simulink model "EV_thermal_charger_2015a_jmaab_Can02"  (R2015a)
settings: Solver=ode3  StartTime=0.0  StopTime=1800  FixedStep=sampling_time  RelTol=1e-3
PreLoadFcn:
  | %run('init_setting.m')
PostLoadFcn:
  | %set_param(gcs, 'SimulationCommand', 'update');
  | %load('save_param/save_P_Charger', 'P_Charger');
  | %load('save_param/save_T_User_set_temp_degC','T_User_set_temp_degC');
  | %load('save_param/save_ENV_PNT_PTTH_Temp_add_degC','ENV_PNT_PTTH_Temp_add_degC');
  | %load('save_param/save_ENV_PNT_CABIN_Temp_add_degC','ENV_PNT_CABIN_Temp_add_degC');
  | %load('save_param/save_ENV_PNT_PHI_Sunlight_W','ENV_PNT_PHI_Sunlight_W');
  | %load('save_param/save_ENV_PNT_Outside_Temp_ini_degC','ENV_PNT_Outside_Temp_ini_degC');
StartFcn:
  | tic
StopFcn:
  | toc
  | disp(['実時間の' num2str(toc/max(tout)) '倍'])
undefined symbols (not defined in the file or in its folder): BK_PNT_Pow_UL, BK_PNT_ReGene_vel_limit_DN_kmph, BK_PNT_ReGene_vel_limit_UP_kmph, BK_PNT_Tau_brake, Brk_LL, Brk_PGain, Brk_UL, BT_PNT_Hi_C_pol_hi_batt, BT_PNT_Hi_Capa_hi_batt_F, BT_PNT_Hi_ocv_SOC_hi_batt_OCV_V_table, BT_PNT_Hi_ocv_SOC_hi_batt_OCV_V_table_x_SOC, BT_PNT_Hi_R_hi_batt_cell, BT_PNT_Hi_R_pol_hi_batt, BT_PNT_Hi_SOC_MAX_hi_batt, BT_PNT_Hi_SOC_MIN_hi_batt, BT_PNT_Hi_SOC_START_hi_batt, BT_PNT_Lo_Capa_lo_batt_F, BT_PNT_Lo_ocv_SOC_lo_batt_OCV_V_table, BT_PNT_Lo_ocv_SOC_lo_batt_OCV_V_table_x_SOC, BT_PNT_Lo_R_lo_batt_ohm, BT_PNT_Lo_SOC_MAX_lo_batt, BT_PNT_Lo_SOC_MIN_lo_batt, BT_PNT_Lo_SOC_START_lo_batt, BTTH_CNT_P_BT_Heater_W, BTTH_CNT_P_BT_Heater_W_x_BTCells_degC, BTTH_CNT_Voltage_BTFan_V, BTTH_CNT_Voltage_BTFan_V_x_BTCells_degC, BTTH_PNT_BT_Heat_Resi_KpW, BTTH_PNT_BT_Heat_Resi_KpW_x_Wind_m3ps, BTTH_PNT_BT_Heater2BTCells_Heat_Resi_KpW, BTTH_PNT_BT_Heater_Heat_Capa_JpK, BTTH_PNT_BTBlock2BTAir_Heat_Resi_KpW, BTTH_PNT_BTBlock_Heat_Capa_JpK, BTTH_PNT_BTCells2BTBlock_Heat_Resi_KpW, BTTH_PNT_BTCells_Heat_Capa_JpK, BTTH_PNT_v_BTFan_Wind_vel_mps, BTTH_PNT_v_BTFan_Wind_vel_mps_x_V_BTFan, CATH_CNT_P_Aircon_W_LL, CATH_CNT_P_Aircon_W_UL, CATH_CNT_P_Gain_Aircon, CATH_CNT_P_Gain_PTC_Heater, CATH_CNT_P_Gain_SeatHT, CATH_CNT_P_PTC_Heater, CATH_CNT_P_PTC_Heater_W_LL, CATH_CNT_P_PTC_Heater_W_UL, CATH_CNT_P_PTC_Heater_x_T_Outside_temp_degC, CATH_CNT_P_SeatHT_W_LL, CATH_CNT_P_SeatHT_W_UL, CATH_CNT_PGain_Temp_blowout, CATH_CNT_T_Aircon_Indoor_degC, CATH_CNT_T_Aircon_Indoor_degC_x_T_blowout_degC, CATH_CNT_T_PTC_Heater_degC_UL, CATH_CNT_T_SeatHT_Temp_degC, CATH_CNT_T_SeatHT_Temp_degC_x_T_blowout_degC, CATH_CNT_V_HVAC_Fan, CATH_CNT_V_HVAC_Fan_x_T_blowout_degC, CATH_CNT_V_RDFan_V, CATH_CNT_V_RDFan_x_P_Aircon_W, CATH_PNT_Air_Convection_Heat_Resi_KpW, CATH_PNT_Air_Convection_Heat_Resi_x_mps ... (+141)
undefined symbols (not defined in the file): ACC_D_Gain, ACC_I_Gain, ACC_P_Gain
libraries: METI_Lib_vehicle_model x52, simulink x35
(part 4 of 6)

== system EV_thermal_charger_2015a_jmaab_Can02/Vehicle/ELTH/ELTH_PNT/INVTH_PNT ==
  note: モーターハウジングへの熱量
  note: ヒートシンクの
      | 熱容量
  note: インバータ筐体の
      | 熱容量
  note: 冷却水からの熱量
  Temp_ini : Inport
  PHI_INV_PNT_W : Inport  Port=2
  T_ATM_PNT_INV_K : Inport  Port=3
  T_MGTH_PNT_INVTH_K : Inport  Port=4
  PHI_RD_PNT_INVTH_W : Inport  Port=5
  INVBlock2Air_Heat_Resistance : Subsystem
  INVBlock_Heat_Capacity : Subsystem
  INVHeatsink2INVBlock_Heat_Resistance : Subsystem
  INVTH_Heatsink_Heat_Capacity : Subsystem
  K->degC1 : Subsystem
  K->degC2 : Subsystem
  MG2INVBlock_Heat_Resistance : Subsystem
  T_INVHeatsink_K : Outport
  T_INVTH_PNT_K : Outport  Port=2
  PHI_INVTH_PNT_ATM_W : Outport  Port=3
  T_INVTH_PNT_RD_K : Outport  Port=4
  PHI_INVTH_PNT_MGTH_W : Outport  Port=5
  tag scope: tScope_T_INVBlock_degC=global, tScope_T_INVHeatsink_degC=global
  wires:
  INVBlock_Heat_Capacity/3(T_INVBlock1_K) -> INVHeatsink2INVBlock_Heat_Resistance/2(T_INVBlock_Resi1_K)
  INVHeatsink2INVBlock_Heat_Resistance/1(PHI_INVBlock_Resi1_W) -> INVBlock_Heat_Capacity/3(PHI_INVBlock1_W)
  INVBlock2Air_Heat_Resistance/2(PHI_INVBlock_Resi3_W) -> INVBlock_Heat_Capacity/4(PHI_INVBlock3_W)
  INVBlock_Heat_Capacity/2(T_INVBlock3_K) -> INVBlock2Air_Heat_Resistance/2(T_INVBlock_Resi3_K), K->degC1/1(K)
  INVBlock2Air_Heat_Resistance/1(PHI_INV2Air_Resi1_W) -> PHI_INVTH_PNT_ATM_W/1  "PHI_INVTH_PNT_ATM_W"
  MG2INVBlock_Heat_Resistance/1(PHI_INVBlock_Resi2_W) -> INVBlock_Heat_Capacity/1(PHI_INVBlock2_W)
  INVBlock_Heat_Capacity/1(T_INVBlock2_K) -> MG2INVBlock_Heat_Resistance/1(T_INVBlock_Resi2_K)
  T_MGTH_PNT_INVTH_K/1 -> MG2INVBlock_Heat_Resistance/2(T_MGBlock_Resi4_K)
  MG2INVBlock_Heat_Resistance/2(PHI_MGBlock_Resi4_W) -> PHI_INVTH_PNT_MGTH_W/1  "HI_INVTH_PNT_MGTH_W"
  INVTH_Heatsink_Heat_Capacity/1(T_INVTH_Heatsink1_K) -> T_INVTH_PNT_K/1  "T_INVTH_PNT_K"
  PHI_INV_PNT_W/1 -> INVTH_Heatsink_Heat_Capacity/2(PHI_INVTH_Heatsink1_W)
  T_ATM_PNT_INV_K/1 -> INVBlock2Air_Heat_Resistance/1(T_INV2Air_Resi1_K)
  INVTH_Heatsink_Heat_Capacity/3(T_INVTH_Heatsink3_K) -> T_INVTH_PNT_RD_K/1, K->degC2/1(K), T_INVHeatsink_K/1  "T_INVHeatsink_K"
  PHI_RD_PNT_INVTH_W/1 -> INVTH_Heatsink_Heat_Capacity/3(PHI_INVTH_Heatsink3_W)
  INVTH_Heatsink_Heat_Capacity/2(T_INVTH_Heatsink2_K) -> INVHeatsink2INVBlock_Heat_Resistance/1(T_INVHeatsink_Resi2_K)
  INVHeatsink2INVBlock_Heat_Resistance/2(PHI_INVHeatsink_Resi2_W) -> INVTH_Heatsink_Heat_Capacity/4(PHI_INVTH_Heatsink2_W)
  Temp_ini/1 -> INVTH_Heatsink_Heat_Capacity/1(Temp_ini), INVBlock_Heat_Capacity/2(Temp_ini)
  K->degC2/1(degC) -> [tScope_T_INVHeatsink_degC]
  K->degC1/1(degC) -> [tScope_T_INVBlock_degC]

== system EV_thermal_charger_2015a_jmaab_Can02/Vehicle/ELTH/ELTH_PNT/K->degC1 ==
  K : Inport
  Constant2 : Constant  Value=K2degC
  Sum : Sum  Inputs=++|
  degC : Outport
  wires:
  K/1 -> Sum/2
  Constant2/1 -> Sum/1
  Sum/1 -> degC/1

== system EV_thermal_charger_2015a_jmaab_Can02/Vehicle/ELTH/ELTH_PNT/K->degC3 ==
  K : Inport
  Constant2 : Constant  Value=K2degC
  Sum : Sum  Inputs=++|
  degC : Outport
  wires:
  K/1 -> Sum/2
  Constant2/1 -> Sum/1
  Sum/1 -> degC/1

== system EV_thermal_charger_2015a_jmaab_Can02/Vehicle/ELTH/ELTH_PNT/K->degC6 ==
  K : Inport
  Constant2 : Constant  Value=K2degC
  Sum : Sum  Inputs=++|
  degC : Outport
  wires:
  K/1 -> Sum/2
  Constant2/1 -> Sum/1
  Sum/1 -> degC/1

== system EV_thermal_charger_2015a_jmaab_Can02/Vehicle/ELTH/ELTH_PNT/MGTH_PNT ==
  note: モーターコイルの
      | 熱容量
  note: モーターハウジングの
      | 熱容量
  note: インバータ筐体からの熱量
  note: PTサーマルシステムへの熱量
  note: 冷却水から
      | モーターハウジングへの熱量
  note: モーターの損失が
      | コイルへの熱量
  note: モーターハウジングから大気へ
      | 放熱する熱量
  Temp_ini : Inport
  PHI_MG_PNT_W : Inport  Port=2
  T_TMTH_PNT_ELTH_K : Inport  Port=3
  T_ATM_PNT_MG_K : Inport  Port=4
  " PHI_RD_PNT_MGTH_W" : Inport  Port=5
  PHI_INVTH_PNT_MGTH_W : Inport  Port=6
  Coil_Heat_Capacity : Subsystem
  K->degC1 : Subsystem
  K->degC2 : Subsystem
  MGCoil2MGHousing_Heat_Resistance : Subsystem
  MGHousing2Air_Heat_Resistance : Subsystem
  MGHousing_Heat_Capacity : Subsystem
  PTTH2MGHousing_Heat_Resistance : Subsystem
  T_MGCoil_K : Outport
  T_MGTH_PNT_K : Outport  Port=2
  PHI_MGTH_PNT_PTTH_W : Outport  Port=3
  PHI_MGTH_PNT_ATM_W : Outport  Port=4
  T_MGTH_PNT_RD_K : Outport  Port=5
  T_MGTH_PNT_INVTH_K : Outport  Port=6
  tag scope: tScope_T_MGBlock_degC=global, tScope_T_MGCoil_degC=global
  wires:
  Coil_Heat_Capacity/2(T_MGCoil2_K) -> MGCoil2MGHousing_Heat_Resistance/1(T_MGCoil_Resi4_K), K->degC1/1(K)
  MGCoil2MGHousing_Heat_Resistance/2(PHI_MGCoil_Resi4_W) -> Coil_Heat_Capacity/3(PHI_MGCoil2_W)
  MGHousing_Heat_Capacity/5(T_MGHousing1_K) -> MGCoil2MGHousing_Heat_Resistance/2(T_MGHousing_Resi1_K)
  Coil_Heat_Capacity/1(T_MGCoil1_K) -> T_MGTH_PNT_K/1, T_MGCoil_K/1  "T_MGTH_PNT_K"
  PHI_MG_PNT_W/1 -> Coil_Heat_Capacity/2(PHI_MGCoil1_W)
  T_TMTH_PNT_ELTH_K/1 -> PTTH2MGHousing_Heat_Resistance/2(T_PTTH_Resi2_K)
  PTTH2MGHousing_Heat_Resistance/2(PHI_PTTH_Resi2_W) -> PHI_MGTH_PNT_PTTH_W/1  "PHI_MGTH_PNT_PTTH_W"
  PTTH2MGHousing_Heat_Resistance/1(PHI_MGHousing_Resi2_W) -> MGHousing_Heat_Capacity/1(PHI_MGHousing2_W)
  MGHousing_Heat_Capacity/1(T_MGHousing2_K) -> PTTH2MGHousing_Heat_Resistance/1(T_MGHousing_Resi2_K)
  T_ATM_PNT_MG_K/1 -> MGHousing2Air_Heat_Resistance/1(T_MG2Air_Resi1_K)
  MGHousing2Air_Heat_Resistance/1(PHI_MG2Air_Resi1_W) -> PHI_MGTH_PNT_ATM_W/1  "PHI_MGTH_PNT_ATM_W"
  MGHousing_Heat_Capacity/3(T_MGHousing4_K) -> T_MGTH_PNT_INVTH_K/1  "T_MGTH_PNT_INVTH_K"
  PHI_INVTH_PNT_MGTH_W/1 -> MGHousing_Heat_Capacity/3(PHI_MGHousing4_W)
  MGHousing_Heat_Capacity/4(T_MGHousing5_K) -> K->degC2/1(K), MGHousing2Air_Heat_Resistance/2(T_MGHousing_Resi5_K)
  MGHousing2Air_Heat_Resistance/2(PHI_MGHousing_Resi5_W) -> MGHousing_Heat_Capacity/6(PHI_MGHousing5_W)
  MGHousing_Heat_Capacity/2(T_MGHousing3_K) -> T_MGTH_PNT_RD_K/1  "T_MGTH_PNT_RD_K"
  " PHI_RD_PNT_MGTH_W"/1 -> MGHousing_Heat_Capacity/2(PHI_MGHousing3_W)
  Temp_ini/1 -> Coil_Heat_Capacity/1(Temp_ini), MGHousing_Heat_Capacity/4(Temp_ini)
  K->degC1/1(degC) -> [tScope_T_MGCoil_degC]
  K->degC2/1(degC) -> [tScope_T_MGBlock_degC]
  MGCoil2MGHousing_Heat_Resistance/1(PHI_MGHousing_Resi1_W) -> MGHousing_Heat_Capacity/5(PHI_MGHousing1_W)

== system EV_thermal_charger_2015a_jmaab_Can02/Vehicle/ELTH/ELTH_PNT/RD_PNT ==
  note: ラジエター～大気間
      | 熱抵抗
  note: 冷却水＋ラジエターコア
      | 熱容量
  Temp_ini : Inport
  v_VL_PNT_mps : Inport  Port=2
  V_ELTH_CNT_RDFan_V : Inport  Port=3
  V_ELTH_CNT_WP_V : Inport  Port=4
  T_ATM_PNT_RD_K : Inport  Port=5
  T_MGTH_PNT_RD_K : Inport  Port=6
  T_INVTH_PNT_RD_K : Inport  Port=7
  Add : Sum
  INV2Coolant_Heat_Resistance1 : Subsystem
  K->degC1 : Subsystem
  MG2Coolant_Heat_Resistance : Subsystem
  RDCoolant2Air_Heat_Resistance : Subsystem
  RDCoolant_Heat_Capacity : Subsystem
  RD_Core_Heat_Resi_Calc : Subsystem
  Water_Pump : Subsystem
  T_RDCoolant_K : Outport
  Heat_Resi_ELTH_PNT_AirconCore_KpW : Outport  Port=2
  PHI_RDTH_PNT_ATM_W : Outport  Port=3
  PHI_RD_PNT_MGTH_W : Outport  Port=4
  PHI_RD_PNT_INVTH_W : Outport  Port=5
  tag scope: tScope_T_RDCoolant_degC=global
  wires:
  RDCoolant_Heat_Capacity/2(T_RDCoolant1_K) -> INV2Coolant_Heat_Resistance1/3(T_Coolant_Resi_K)
  INV2Coolant_Heat_Resistance1/1(PHI_Coolant_Resi_W) -> RDCoolant_Heat_Capacity/2(PHI_RDCoolant1_W)
  RDCoolant2Air_Heat_Resistance/1(PHI_RD_Air_Resi1_W) -> PHI_RDTH_PNT_ATM_W/1  "PHI_RDTH_PNT_ATM_W"
  RDCoolant2Air_Heat_Resistance/2(PHI_RDCoolant_Resi2_W) -> RDCoolant_Heat_Capacity/3(PHI_RDCoolant2_W)
  V_ELTH_CNT_RDFan_V/1 -> RD_Core_Heat_Resi_Calc/1(ELTH_PNT_Voltage_RDFan_V)
  v_VL_PNT_mps/1 -> RD_Core_Heat_Resi_Calc/2(v_VL_PNT_mps)
  RD_Core_Heat_Resi_Calc/1("ELTH_PNT_RDCore_Heat_Resi_KpW ") -> RDCoolant2Air_Heat_Resistance/2("RD_PNT_RDCore_Heat_Resi_KpW ")
  T_ATM_PNT_RD_K/1 -> RDCoolant2Air_Heat_Resistance/1(T_RD_Air_Resi1_K)
  RDCoolant_Heat_Capacity/1(T_RDCoolant2_K) -> T_RDCoolant_K/1, K->degC1/1(K), RDCoolant2Air_Heat_Resistance/3(T_RDCoolant_Resi2_K)  "T_RDCoolant_K"
  Water_Pump/1(Qv_Coolant_m3ps) -> MG2Coolant_Heat_Resistance/2(Qv_Coolant_m3ps), INV2Coolant_Heat_Resistance1/1(Qv_Coolant_m3ps)
  T_MGTH_PNT_RD_K/1 -> MG2Coolant_Heat_Resistance/3(T_MGTH_Resi2_K)
  MG2Coolant_Heat_Resistance/1(PHI_MGTH_Resi2_W) -> PHI_RD_PNT_MGTH_W/1
  T_INVTH_PNT_RD_K/1 -> MG2Coolant_Heat_Resistance/1(T_Coolant_Resi2_K), INV2Coolant_Heat_Resistance1/2(T_INVTH_Resi_K)
  Add/1 -> PHI_RD_PNT_INVTH_W/1  "PHI_RD_PNT_INVTH_W"
  INV2Coolant_Heat_Resistance1/2(PHI_INVTH_Resi_W) -> Add/1
  MG2Coolant_Heat_Resistance/2(PHI_Coolant_Resi2_W) -> Add/2
  V_ELTH_CNT_WP_V/1 -> Water_Pump/1(ELTH_PNT_Voltage_WP_V)
  Temp_ini/1 -> RDCoolant_Heat_Capacity/1(Temp_ini)
  RD_Core_Heat_Resi_Calc/2(ELTH_PNT_AirconCore_Heat_Resi_KpW) -> Heat_Resi_ELTH_PNT_AirconCore_KpW/1  "Heat_Resi_ELTH_PNT_AirconCore_KpW"
  K->degC1/1(degC) -> [tScope_T_RDCoolant_degC]

== system EV_thermal_charger_2015a_jmaab_Can02/Vehicle/INV_PT/INV_PNT/Divide_0wari1 ==
  ÷ : Inport
  × : Inport  Port=2
  Constant : Constant  Value=0
  Constant1 : Constant
  Constant2 : Constant  Value=0
  Divide : Product  Inputs=*/
  Logical Operator : Logic  Operator=OR  AllPortsSameDT=off  OutDataTypeStr=boolean
  Relational Operator : RelationalOperator  Operator=>  OutDataTypeStr=boolean
  Relational Operator1 : RelationalOperator  Operator=<  OutDataTypeStr=boolean
  Switch : Switch  Criteria=u2 > Threshold  Threshold=0.5
  Switch1 : Switch  Criteria=u2 > Threshold  Threshold=0.5
  "　" : Outport
  wires:
  Switch1/1 -> "　"/1
  Constant2/1 -> Switch1/3
  Constant1/1 -> Switch/3
  Logical Operator/1 -> Switch/2, Switch1/2
  Switch/1 -> Divide/2
  Relational Operator1/1 -> Logical Operator/2
  Relational Operator/1 -> Logical Operator/1
  Constant/1 -> Relational Operator/2, Relational Operator1/2
  ÷/1 -> Switch/1, Relational Operator/1, Relational Operator1/1
  Divide/1 -> Switch1/1
  ×/1 -> Divide/1

== system EV_thermal_charger_2015a_jmaab_Can02/Vehicle/INV_PT/INV_PNT/Divide_0wari2 ==
  ÷ : Inport
  × : Inport  Port=2
  Constant : Constant  Value=0
  Constant1 : Constant
  Constant2 : Constant  Value=0
  Divide : Product  Inputs=*/
  Logical Operator : Logic  Operator=OR  AllPortsSameDT=off  OutDataTypeStr=boolean
  Relational Operator : RelationalOperator  Operator=>  OutDataTypeStr=boolean
  Relational Operator1 : RelationalOperator  Operator=<  OutDataTypeStr=boolean
  Switch : Switch  Criteria=u2 > Threshold  Threshold=0.5
  Switch1 : Switch  Criteria=u2 > Threshold  Threshold=0.5
  "　" : Outport
  wires:
  Switch1/1 -> "　"/1
  Constant2/1 -> Switch1/3
  Constant1/1 -> Switch/3
  Logical Operator/1 -> Switch/2, Switch1/2
  Switch/1 -> Divide/2
  Relational Operator1/1 -> Logical Operator/2
  Relational Operator/1 -> Logical Operator/1
  Constant/1 -> Relational Operator/2, Relational Operator1/2
  ÷/1 -> Switch/1, Relational Operator/1, Relational Operator1/1
  Divide/1 -> Switch1/1
  ×/1 -> Divide/1

== system EV_thermal_charger_2015a_jmaab_Can02/Vehicle/INV_PT/INV_PNT/Subsystem ==
  eta : Inport
  OUT_Power : Inport  Port=2
  Constant : Constant
  Product : Product  Inputs=*/
  Product1 : Product
  Saturation : Saturate  UpperLimit=1  LowerLimit=-1
      settings: AttributesFormatString=%<LowerLimit> < u < %<UpperLimit>
  Sum1 : Sum  Inputs=|-+
  Switch : Switch  Criteria=u2 > Threshold
  Loss_Power : Outport
  IN_Power : Outport  Port=2
  wires:
  Sum1/1 -> Loss_Power/1
  Saturation/1 -> Switch/2
  eta/1 -> Switch/3, Product/2
  Constant/1 -> Product/1
  Switch/1 -> Product1/2
  OUT_Power/1 -> Sum1/1, Product1/1, Saturation/1
  Product1/1 -> Sum1/2, IN_Power/1
  Product/1 -> Switch/1

== system EV_thermal_charger_2015a_jmaab_Can02/Vehicle/MG_PNT/MG_PNT/Power_Conversion ==
  note: U相電流
  note: U-V線間電圧
  note: U相有効電圧
  note: UVW三相合計の
      | モータートルク
  note: U相皮相電圧
  k_MG_CNT_Vpradps : Inport
  Power_factor_INV_PNT : Inport  Port=2
  "w_TM_PNT_radps " : Inport  Port=3
  "I_INV_PNT_AC_A " : Inport  Port=4
  Constant1 : Constant  Value=3
  Constant2 : Constant  Value=sqrt(3)
  Divide : Product  Inputs=/*
  Product{,1,3..4} (4 alike) : Product
  V_MG_PNT_AC_V : Outport
  "trq_Power_Conversion_Nm " : Outport  Port=2
  wires:
  k_MG_CNT_Vpradps/1 -> Product1/1, Product/2
  Product1/1 -> "trq_Power_Conversion_Nm "/1  "trq_UPhase"
  Divide/1 -> Product4/1
  Product3/1 -> Product1/2
  Constant2/1 -> Product4/2
  Constant1/1 -> Product3/1
  "I_INV_PNT_AC_A "/1 -> Product3/2
  Power_factor_INV_PNT/1 -> Divide/1
  Product/1 -> Divide/2
  "w_TM_PNT_radps "/1 -> Product/1
  Product4/1 -> V_MG_PNT_AC_V/1  "V_MG_PNT_AC_V"

== system EV_thermal_charger_2015a_jmaab_Can02/Vehicle/BAT_Hi_PNT/BT_Hi_PNT/Cal_SOC/Subsystem4 ==
  In1 : Inport
  In2 : Inport  Port=2
  To Workspace : ToWorkspace  VariableName=SOC_LoBat  SampleTime=-1
      settings: Decimation=num_tws_mabiki
  To Workspace1 : ToWorkspace  VariableName=Asec_LoBat  SampleTime=-1
      settings: Decimation=num_tws_mabiki
  wires:
  In1/1 -> To Workspace/1
  In2/1 -> To Workspace1/1

== system EV_thermal_charger_2015a_jmaab_Can02/Vehicle/BTTH/BTTH_PNT/BB_PNT/BTBlock_Heat_Capacity ==
  ini_T_Environment_Outside_degC : Inport
  PHI_BTBlock1_W : Inport  Port=2
  PHI_BTBlock2_W : Inport  Port=3
  Add : Sum
  Add1 : Sum
  Constant : Constant  Value=BTTH_PNT_BTBlock_Heat_Capa_JpK
  Divide : Product  Inputs=/*
  Integrator : Integrator
  degC->K : Subsystem
  T_BTBlock1_K : Outport
  T_BTBlock2_K : Outport  Port=2
  wires:
  PHI_BTBlock2_W/1 -> Add/2
  PHI_BTBlock1_W/1 -> Add/1
  Constant/1 -> Divide/1
  Add/1 -> Divide/2
  Divide/1 -> Integrator/1
  ini_T_Environment_Outside_degC/1 -> degC->K/1(degC)
  Integrator/1 -> Add1/2
  Add1/1 -> T_BTBlock1_K/1, T_BTBlock2_K/1
  degC->K/1(K) -> Add1/1

== system EV_thermal_charger_2015a_jmaab_Can02/Vehicle/BTTH/BTTH_PNT/BB_PNT/BT_Block2Air_Heat_Resistance ==
  T_ATM_PNT_BB_K : Inport
  T_BTBlock_Resi2_K : Inport  Port=2
  Add : Sum  Inputs=+-
  Constant : Constant  Value=BTTH_PNT_BTBlock2BTAir_Heat_Resi_KpW
  Divide : Product  Inputs=*/
  Gain : Gain  Gain=-1
  Gain1 : Gain
  PHI_BT2AIR_Resi1_W : Outport
  PHI_BTBlock_Resi2_W : Outport  Port=2
  wires:
  Constant/1 -> Divide/2
  Add/1 -> Divide/1
  Divide/1 -> Gain/1, Gain1/1
  Gain/1 -> PHI_BTBlock_Resi2_W/1
  T_BTBlock_Resi2_K/1 -> Add/1
  T_ATM_PNT_BB_K/1 -> Add/2
  Gain1/1 -> PHI_BT2AIR_Resi1_W/1

== system EV_thermal_charger_2015a_jmaab_Can02/Vehicle/BTTH/BTTH_PNT/BC_PNT/BTCells_Heat_Capacity ==
  ini_T_Environment_Outside_degC : Inport
  PHI_BTCells1_W : Inport  Port=2
  PHI_BTCells2_W : Inport  Port=3
  PHI_BTCells3_W : Inport  Port=4
  PHI_BTCells4_W : Inport  Port=5
  Add : Sum  Inputs=++++
  Add1 : Sum
  Constant : Constant  Value=BTTH_PNT_BTCells_Heat_Capa_JpK
  Divide : Product  Inputs=/*
  Integrator : Integrator
  degC->K : Subsystem
  T_BTCells1_K : Outport
  T_BTCells2_K : Outport  Port=2
  T_BTCells3_K : Outport  Port=3
  T_BTCells4_K : Outport  Port=4
  wires:
  PHI_BTCells1_W/1 -> Add/1
  Constant/1 -> Divide/1
  Add/1 -> Divide/2
  Divide/1 -> Integrator/1
  ini_T_Environment_Outside_degC/1 -> degC->K/1(degC)
  Integrator/1 -> Add1/2
  Add1/1 -> T_BTCells4_K/1, T_BTCells3_K/1, T_BTCells1_K/1, T_BTCells2_K/1
  degC->K/1(K) -> Add1/1
  PHI_BTCells2_W/1 -> Add/2
  PHI_BTCells3_W/1 -> Add/3
  PHI_BTCells4_W/1 -> Add/4

== system EV_thermal_charger_2015a_jmaab_Can02/Vehicle/BTTH/BTTH_PNT/BC_PNT/BT_Cells2BTBlock_Heat_Resistance ==
  T_BTBlock_Resi1_K : Inport
  T_BTCells_Resi2_K : Inport  Port=2
  Add : Sum  Inputs=+-
  Constant : Constant  Value=BTTH_PNT_BTCells2BTBlock_Heat_Resi_KpW
  Divide : Product  Inputs=*/
  Gain : Gain  Gain=-1
  Gain1 : Gain
  PHI_BTBlock_Resi1_W : Outport
  PHI_BTCells_Resi2_W : Outport  Port=2
  wires:
  Constant/1 -> Divide/2
  Add/1 -> Divide/1
  Divide/1 -> Gain/1, Gain1/1
  T_BTCells_Resi2_K/1 -> Add/1
  T_BTBlock_Resi1_K/1 -> Add/2
  Gain1/1 -> PHI_BTBlock_Resi1_W/1
  Gain/1 -> PHI_BTCells_Resi2_W/1

== system EV_thermal_charger_2015a_jmaab_Can02/Vehicle/BTTH/BTTH_PNT/BF_PNT/BTFan_Heat_Resistance ==
  "BTTH_PNT_BTFan_Heat_Resi_KpW " : Inport
  T_ATM_PNT_BF_K : Inport  Port=2
  T_BT_Fan_Resi2_K : Inport  Port=3
  Add : Sum  Inputs=+-
  Divide : Product  Inputs=*/
  Gain : Gain  Gain=-1
  Gain1 : Gain
  PHI_BT_Fan_Resi1_W : Outport
  PHI_BT_Fan_Resi2_W : Outport  Port=2
  wires:
  "BTTH_PNT_BTFan_Heat_Resi_KpW "/1 -> Divide/2
  Add/1 -> Divide/1
  Divide/1 -> Gain/1, Gain1/1
  Gain/1 -> PHI_BT_Fan_Resi2_W/1
  T_BT_Fan_Resi2_K/1 -> Add/1
  T_ATM_PNT_BF_K/1 -> Add/2
  Gain1/1 -> PHI_BT_Fan_Resi1_W/1

== system EV_thermal_charger_2015a_jmaab_Can02/Vehicle/BTTH/BTTH_PNT/BF_PNT/BT_Fan_Heat_Resi_Calc ==
  note: ラジエターファンの動作で
      | 発生する風速
  BTTH_PNT_Voltage_BTFan_V : Inport
  1-D Lookup Table : Lookup_n-D  NumberOfTableDimensions=1  BreakpointsForDimension1=BTTH_PNT_BT_Heat_Resi_KpW_x_Wind_m3ps  Table=BTTH_PNT_BT_Heat_Resi_KpW  InternalRulePriority=Speed  RndMeth=Simplest  InputSameDT=on
  1-D Lookup Table1 : Lookup_n-D  NumberOfTableDimensions=1  BreakpointsForDimension1=BTTH_PNT_v_BTFan_Wind_vel_mps_x_V_BTFan  Table=BTTH_PNT_v_BTFan_Wind_vel_mps  InternalRulePriority=Speed  RndMeth=Simplest  InputSameDT=on
  "BTTH_PNT_BTFan_Heat_Resi_KpW " : Outport
  wires:
  BTTH_PNT_Voltage_BTFan_V/1 -> 1-D Lookup Table1/1
  1-D Lookup Table/1 -> "BTTH_PNT_BTFan_Heat_Resi_KpW "/1
  1-D Lookup Table1/1 -> 1-D Lookup Table/1

== system EV_thermal_charger_2015a_jmaab_Can02/Vehicle/BTTH/BTTH_PNT/BH_PNT/BT_Heater ==
  T_BT_Heater_K : Inport
  tgt_P_BTTH_CNT_BTHeater_W : Inport  Port=2
  V_BT_Lo_PNT_V : Inport  Port=3
  Divide_0wari : METI_Lib_vehicle_model/Divide_0wari
  Gain : Gain  Gain=-1
  Terminator : Terminator
  PHI_BT_Heater_W : Outport
  I_BT_Heater_A : Outport  Port=2
  wires:
  Divide_0wari/1 -> Gain/1
  tgt_P_BTTH_CNT_BTHeater_W/1 -> PHI_BT_Heater_W/1, Divide_0wari/1
  V_BT_Lo_PNT_V/1 -> Divide_0wari/2
  T_BT_Heater_K/1 -> Terminator/1
  Gain/1 -> I_BT_Heater_A/1

== system EV_thermal_charger_2015a_jmaab_Can02/Vehicle/BTTH/BTTH_PNT/BH_PNT/BT_Heater2BTCells_Heat_Resistance ==
  T_BTCells_Resi1_K : Inport
  T_BT_Heater_Resi2_K : Inport  Port=2
  Add : Sum  Inputs=+-
  Constant : Constant  Value=BTTH_PNT_BT_Heater2BTCells_Heat_Resi_KpW
  Divide : Product  Inputs=*/
  Gain : Gain  Gain=-1
  Gain1 : Gain
  PHI_BTCells_Resi1_W : Outport
  PHI_BT_Heater_Resi2_W : Outport  Port=2
  wires:
  Constant/1 -> Divide/2
  Add/1 -> Divide/1
  Divide/1 -> Gain/1, Gain1/1
  Gain/1 -> PHI_BT_Heater_Resi2_W/1
  T_BT_Heater_Resi2_K/1 -> Add/1
  T_BTCells_Resi1_K/1 -> Add/2
  Gain1/1 -> PHI_BTCells_Resi1_W/1

== system EV_thermal_charger_2015a_jmaab_Can02/Vehicle/BTTH/BTTH_PNT/BH_PNT/BT_Heater_Heat_Capacity ==
  PHI_BTCells_Resi1_W : Inport
  PHI_BT_Heater1_W : Inport  Port=2
  PHI_BT_Heater2_W : Inport  Port=3
  Add : Sum
  Add1 : Sum
  Constant : Constant  Value=BTTH_PNT_BT_Heater_Heat_Capa_JpK
  Divide : Product  Inputs=/*
  Integrator : Integrator
  degC->K : Subsystem
  T_BT_Heater1_K : Outport
  T_BT_Heater2_K : Outport  Port=2
  wires:
  PHI_BT_Heater2_W/1 -> Add/2
  PHI_BT_Heater1_W/1 -> Add/1
  Constant/1 -> Divide/1
  Add/1 -> Divide/2
  Divide/1 -> Integrator/1
  PHI_BTCells_Resi1_W/1 -> degC->K/1(degC)
  Integrator/1 -> Add1/2
  Add1/1 -> T_BT_Heater2_K/1, T_BT_Heater1_K/1
  degC->K/1(K) -> Add1/1

== system EV_thermal_charger_2015a_jmaab_Can02/Vehicle/CATH/CATH_PNT/CABIN/CABIN_AIR ==
  note: 車室空気の
      | 熱容量
  note: ヒートポンプからの
      | 熱量
  note: PTCヒータからの
      | 熱量
  note: シートヒータからの
      | 熱量
  note: 直射日光からの
      | 熱量
  note: ガラスを通した
      | 外気からの熱量
  note: 不透明壁からの
      | 赤外線輻射による熱量
  note: 不透明壁を通した
      | 外気からの熱量
  note: 乗員からの
      | 熱量
  Temp_ini1 : Inport
  PHI_CABIN_Aircon_W : Inport  Port=2
  PHI_CABIN_PTC_W : Inport  Port=3
  PHI_CABIN_SeatHT_W : Inport  Port=4
  PHI_CABIN_Human_W : Inport  Port=5
  PHI_CABIN_Sunlight_W : Inport  Port=6
  PHI_CABIN_Glass_W : Inport  Port=7
  PHI_CABIN_Wall_W : Inport  Port=8
  PHI_CABIN_Radiation_W : Inport  Port=9
  Add : Sum  Inputs=++++++++
  Add1 : Sum
  Constant : Constant  Value=CATH_PNT_CABIN_AIR_Heat_Capa_JpK
  Divide : Product  Inputs=/*
  Integrator : Integrator  LowerSaturationLimit=0
  degC->K : Subsystem
  T_CABIN_AIR_temp_K1 : Outport
  T_CABIN_Aicon_K : Outport  Port=2
  T_CABIN_PTC_K : Outport  Port=3
  T_CABIN_SeatHT_K : Outport  Port=4
  T_CABIN_Glass_K : Outport  Port=5
  T_CABIN_Sunlight_K : Outport  Port=6
  T_CABIN_Wall_K : Outport  Port=7
  T_CABIN_Radiation_K : Outport  Port=8
  T_CABIN_Human_K : Outport  Port=9
  wires:
  Add1/1 -> T_CABIN_Aicon_K/1, T_CABIN_PTC_K/1, T_CABIN_SeatHT_K/1, T_CABIN_Human_K/1, T_CABIN_Wall_K/1, T_CABIN_Radiation_K/1, T_CABIN_Glass_K/1, T_CABIN_Sunlight_K/1, T_CABIN_AIR_temp_K1/1
  Constant/1 -> Divide/1
  Add/1 -> Divide/2
  Divide/1 -> Integrator/1
  Temp_ini1/1 -> degC->K/1(degC)
  Integrator/1 -> Add1/2
  degC->K/1(K) -> Add1/1
  PHI_CABIN_Aircon_W/1 -> Add/1
  PHI_CABIN_PTC_W/1 -> Add/2
  PHI_CABIN_SeatHT_W/1 -> Add/3
  PHI_CABIN_Human_W/1 -> Add/4
  PHI_CABIN_Wall_W/1 -> Add/5
  PHI_CABIN_Radiation_W/1 -> Add/6
  PHI_CABIN_Glass_W/1 -> Add/7
  PHI_CABIN_Sunlight_W/1 -> Add/8

== system EV_thermal_charger_2015a_jmaab_Can02/Vehicle/CATH/CATH_PNT/CABIN/GLASS ==
  note: 室内の風速
  V_vehicle_mps : Inport
  Temp_ini : Inport  Port=2
  T_GLASS2AIR_K : Inport  Port=3
  PHI_GLASS_Sunlight2_W : Inport  Port=4
  T_GLASS_CABIN_K : Inport  Port=5
  T_GLASS_Sunlight1_K : Inport  Port=6
  CABIN_Glass_Heat_Capacity : Subsystem
  CABIN_Glass_Heat_Resistance : Subsystem
  CABIN_Glass_Heat_Resistance1 : Subsystem
  Constant : Constant  Value=5
  PHI_GLASS2AIR_W : Outport
  T_GLASS_Sunlight2_K : Outport  Port=2
  PHI_GLASS_Sunlight1_W : Outport  Port=3
  PHI_GLASS_CABIN_W : Outport  Port=4
  wires:
  CABIN_Glass_Heat_Resistance/1(PHI_CABIN_Glass_Resi1_W) -> PHI_GLASS2AIR_W/1
  T_GLASS2AIR_K/1 -> CABIN_Glass_Heat_Resistance/2(T_CABIN_Glass_Resi1_K)
  CABIN_Glass_Heat_Capacity/2(T_CABIN_Glass1_K) -> CABIN_Glass_Heat_Resistance1/3(T_CABIN_Glass_Resi3_K)
  CABIN_Glass_Heat_Resistance1/2(PHI_CABIN_Glass_Resi3_W) -> CABIN_Glass_Heat_Capacity/2(PHI_CABIN_Glass1_W)
  CABIN_Glass_Heat_Capacity/1(T_CABIN_Glass2_K) -> CABIN_Glass_Heat_Resistance/3(T_CABIN_Glass_Resi2_K)
  CABIN_Glass_Heat_Resistance/2(PHI_CABIN_Glass_Resi2_W) -> CABIN_Glass_Heat_Capacity/3(PHI_CABIN_Glass2_W)
  PHI_GLASS_Sunlight2_W/1 -> PHI_GLASS_Sunlight1_W/1
  T_GLASS_Sunlight1_K/1 -> T_GLASS_Sunlight2_K/1
  Temp_ini/1 -> CABIN_Glass_Heat_Capacity/1(Temp_ini)
  T_GLASS_CABIN_K/1 -> CABIN_Glass_Heat_Resistance1/2(T_CABIN_Glass_Resi4_K)
  CABIN_Glass_Heat_Resistance1/1(PHI_CABIN_Glass_Resi4_W) -> PHI_GLASS_CABIN_W/1
  Constant/1 -> CABIN_Glass_Heat_Resistance1/1(V_wind)
  V_vehicle_mps/1 -> CABIN_Glass_Heat_Resistance/1(V_wind)

== system EV_thermal_charger_2015a_jmaab_Can02/Vehicle/CATH/CATH_PNT/CABIN/Human_Thermal ==
  T_Human_Thermal_K : Inport
  Constant : Constant  Value=CATH_PNT_PHI_Human_body_W
  Terminator : Terminator
  PHI_Human_Thermal_W : Outport
  wires:
  Constant/1 -> PHI_Human_Thermal_W/1
  T_Human_Thermal_K/1 -> Terminator/1

== system EV_thermal_charger_2015a_jmaab_Can02/Vehicle/CATH/CATH_PNT/CABIN/K->degC ==
  K : Inport
  Constant2 : Constant  Value=K2degC
  Sum : Sum  Inputs=++|
  degC : Outport
  wires:
  K/1 -> Sum/2
  Constant2/1 -> Sum/1
  Sum/1 -> degC/1

== system EV_thermal_charger_2015a_jmaab_Can02/Vehicle/CATH/CATH_PNT/CABIN/K->degC1 ==
  K : Inport
  Constant2 : Constant  Value=K2degC
  Sum : Sum  Inputs=++|
  degC : Outport
  wires:
  K/1 -> Sum/2
  Constant2/1 -> Sum/1
  Sum/1 -> degC/1

== system EV_thermal_charger_2015a_jmaab_Can02/Vehicle/CATH/CATH_PNT/CABIN/K->degC2 ==
  K : Inport
  Constant2 : Constant  Value=K2degC
  Sum : Sum  Inputs=++|
  degC : Outport
  wires:
  K/1 -> Sum/2
  Constant2/1 -> Sum/1
  Sum/1 -> degC/1

== system EV_thermal_charger_2015a_jmaab_Can02/Vehicle/CATH/CATH_PNT/CABIN/K->degC3 ==
  K : Inport
  Constant2 : Constant  Value=K2degC
  Sum : Sum  Inputs=++|
  degC : Outport
  wires:
  K/1 -> Sum/2
  Constant2/1 -> Sum/1
  Sum/1 -> degC/1

== system EV_thermal_charger_2015a_jmaab_Can02/Vehicle/CATH/CATH_PNT/CABIN/WALL ==
  note: 室内の風速
  V_vehicle_mps : Inport
  Temp_ini : Inport  Port=2
  T_WALL2AIR_K : Inport  Port=3
  PHI_WALL_Radiation_W : Inport  Port=4
  T_WALL_CABIN_K : Inport  Port=5
  T_WALL_Radiation1_K : Inport  Port=6
  CABIN_Wall_Heat_Capacity : Subsystem
  CABIN_Wall_Heat_Resistance : Subsystem
  CABIN_Wall_Heat_Resistance1 : Subsystem
  Constant1 : Constant  Value=5
  PHI_WALL2AIR_W : Outport
  T_WALL_Radiation_K : Outport  Port=2
  PHI_WALL_CABIN_W : Outport  Port=3
  PHI_WALL_Radiation1_W : Outport  Port=4
  wires:
  CABIN_Wall_Heat_Resistance/1(PHI_Wall_Resi1_W) -> PHI_WALL2AIR_W/1
  T_WALL2AIR_K/1 -> CABIN_Wall_Heat_Resistance/2(T_Wall_Resi1_K)
  CABIN_Wall_Heat_Capacity/2(T_CABIN_Wall1_K) -> CABIN_Wall_Heat_Resistance1/3(T_CABIN_Wall_Resi1_K)
  CABIN_Wall_Heat_Resistance1/2(PHI_CABIN_Wall_Resi1_W) -> CABIN_Wall_Heat_Capacity/2(PHI_CABIN_Wall1_W)
  CABIN_Wall_Heat_Capacity/1(T_CABIN_Wall2_K) -> CABIN_Wall_Heat_Resistance/3(T_Wall_Resi2_K)
  CABIN_Wall_Heat_Resistance/2(PHI_Wall_Resi2_W) -> CABIN_Wall_Heat_Capacity/3(PHI_CABIN_Wall2_W)
  Temp_ini/1 -> CABIN_Wall_Heat_Capacity/1(Temp_ini)
  T_WALL_CABIN_K/1 -> CABIN_Wall_Heat_Resistance1/2(T_CABIN_Wall_Resi2_K)
  CABIN_Wall_Heat_Resistance1/1(PHI_CABIN_Wall_Resi2_W) -> PHI_WALL_CABIN_W/1
  Constant1/1 -> CABIN_Wall_Heat_Resistance1/1(V_wind)
  V_vehicle_mps/1 -> CABIN_Wall_Heat_Resistance/1(V_wind)
  T_WALL_Radiation1_K/1 -> T_WALL_Radiation_K/1
  PHI_WALL_Radiation_W/1 -> PHI_WALL_Radiation1_W/1

== system EV_thermal_charger_2015a_jmaab_Can02/Vehicle/CATH/CATH_PNT/HVAC/Aircon ==
  note: 室外機の
      | 熱容量
  note: 室内機の
      | 熱容量
  P_Heatpomp_Power : Inport
  Temp_ini : Inport  Port=2
  V_Aircon_V : Inport  Port=3
  PHI_Aircon_Outdoor1_W : Inport  Port=4
  PHI_Aircon_Indoor1_W : Inport  Port=5
  Aircon_Indoor_Unit_Heat_Capacity1 : Subsystem
  Aircon_Outdoor_Unit_Heat_Capacity : Subsystem
  Gain1 : Gain  Gain=-1
  K->degC : Subsystem
  K->degC1 : Subsystem
  Product1 : Product
  Switching_Air_Conditioning_Circuit : Subsystem
  T_Aircon_Outdoor_degC : Outport
  T_Aircon_Indoor_degC : Outport  Port=2
  T_Aircon_Outdoor1_K : Outport  Port=3
  T_Aircon_Indoor1_K : Outport  Port=4
  I_Aircon_A : Outport  Port=5
  tag scope: tScope_PHI_Aircon_Indoor1=global, tScope_PHI_Aircon_Outdoor1=global, tScope_P_Aircon=global
  wires:
  Aircon_Indoor_Unit_Heat_Capacity1/1(T_Aircon_Indoor2_K) -> T_Aircon_Indoor1_K/1, K->degC1/1(K)  "T_Aircon_Indoor1_K"
  PHI_Aircon_Indoor1_W/1 -> [tScope_PHI_Aircon_Indoor1], Aircon_Indoor_Unit_Heat_Capacity1/3(PHI_Aircon_Indoor2_W)
  Aircon_Outdoor_Unit_Heat_Capacity/1(T_Aircon_Outdoor2_K) -> T_Aircon_Outdoor1_K/1, K->degC/1(K)  "T_Aircon_Outdoor1_K"
  PHI_Aircon_Outdoor1_W/1 -> Aircon_Outdoor_Unit_Heat_Capacity/3(PHI_Aircon_Outdoor2_W), [tScope_PHI_Aircon_Outdoor1]
  Temp_ini/1 -> Aircon_Outdoor_Unit_Heat_Capacity/1(Temp_ini), Aircon_Indoor_Unit_Heat_Capacity1/1(Temp_ini)
  K->degC/1(degC) -> T_Aircon_Outdoor_degC/1  "T_Aircon_Outdoor_degC"
  K->degC1/1(degC) -> T_Aircon_Indoor_degC/1  "T_Aircon_Indoor_degC"
  Aircon_Outdoor_Unit_Heat_Capacity/2(T_Aircon_Outdoor3_K) -> Switching_Air_Conditioning_Circuit/4(T_Aircon_Outdoor4_K)
  Aircon_Indoor_Unit_Heat_Capacity1/2(T_Aircon_Indoor3_K) -> Switching_Air_Conditioning_Circuit/3(T_Aircon_Indoor4_K)
  P_Heatpomp_Power/1 -> Switching_Air_Conditioning_Circuit/2(P_Heatpomp_Power)
  V_Aircon_V/1 -> Switching_Air_Conditioning_Circuit/1(V_Compressor_V), Product1/1
  Switching_Air_Conditioning_Circuit/1(I_Compressor_A) -> I_Aircon_A/1, Gain1/1
  Product1/1 -> [tScope_P_Aircon]
  Gain1/1 -> Product1/2
  Switching_Air_Conditioning_Circuit/2(PHI_Aircon_Outdoor4_W) -> Aircon_Outdoor_Unit_Heat_Capacity/2(PHI_Aircon_Outdoor3_W)
  Switching_Air_Conditioning_Circuit/3(PHI_Aircon_Indoor4_W) -> Aircon_Indoor_Unit_Heat_Capacity1/2(PHI_Aircon_Indoor3_W)

== system EV_thermal_charger_2015a_jmaab_Can02/Vehicle/CATH/CATH_PNT/HVAC/Aircon_Fan_Heat_Resi_Calc ==
  note: ラジエターファンの動作で
      | ラジエターコアに当たる風量
  CATH_PNT_Voltage_HVAC_Fan_V : Inport
  1-D Lookup Table : Lookup_n-D  NumberOfTableDimensions=1  BreakpointsForDimension1=CATH_PNT_HVAC_Heat_Resi_KpW_x_Wind_m3ps  Table=CATH_PNT_HVAC_Heat_Resi_KpW  InternalRulePriority=Speed  RndMeth=Simplest  InputSameDT=on
  1-D Lookup Table1 : Lookup_n-D  NumberOfTableDimensions=1  BreakpointsForDimension1=CATH_PNT_v_HVAC_Fan_Wind_vel_m3ps_x_V_HVAC_Fan  Table=CATH_PNT_v_HVAC_Fan_Wind_vel_m3ps  InternalRulePriority=Speed  RndMeth=Simplest  InputSameDT=on
  "HVAC_Fan_Heat_Resi_KpW " : Outport
  wires:
  CATH_PNT_Voltage_HVAC_Fan_V/1 -> 1-D Lookup Table1/1
  1-D Lookup Table/1 -> "HVAC_Fan_Heat_Resi_KpW "/1
  1-D Lookup Table1/1 -> 1-D Lookup Table/1

== system EV_thermal_charger_2015a_jmaab_Can02/Vehicle/CATH/CATH_PNT/HVAC/Aircon_Heat_Resistance ==
  "Aircon_Heat_Resi_KpW " : Inport
  T_Aircon_Resi1_K : Inport  Port=2
  T_Aircon_Resi2_K : Inport  Port=3
  Add : Sum  Inputs=+-
  Divide : Product  Inputs=*/
  Gain : Gain  Gain=-1
  Gain1 : Gain
  PHI_Aircon_Resi1_W : Outport
  PHI_Aircon_Resi2_W : Outport  Port=2
  wires:
  "Aircon_Heat_Resi_KpW "/1 -> Divide/2
  Add/1 -> Divide/1
  Divide/1 -> Gain1/1, Gain/1
  Gain/1 -> PHI_Aircon_Resi2_W/1
  T_Aircon_Resi2_K/1 -> Add/1
  T_Aircon_Resi1_K/1 -> Add/2
  Gain1/1 -> PHI_Aircon_Resi1_W/1

== system EV_thermal_charger_2015a_jmaab_Can02/Vehicle/CATH/CATH_PNT/HVAC/Aircon_Heat_Resistance1 ==
  "Aircon_Heat_Resi_KpW " : Inport
  T_Aircon_Resi3_K : Inport  Port=2
  T_Aircon_Resi4_K : Inport  Port=3
  Add : Sum  Inputs=+-
  Divide : Product  Inputs=*/
  Gain : Gain  Gain=-1
  Gain1 : Gain
  PHI_Aircon_Resi3_W : Outport
  PHI_Aircon_Resi4_W : Outport  Port=2
  wires:
  "Aircon_Heat_Resi_KpW "/1 -> Divide/2
  Add/1 -> Divide/1
  Divide/1 -> Gain1/1, Gain/1
  Gain/1 -> PHI_Aircon_Resi4_W/1  "PHI_Aircon_Resi4_W"
  T_Aircon_Resi4_K/1 -> Add/1
  T_Aircon_Resi3_K/1 -> Add/2
  Gain1/1 -> PHI_Aircon_Resi3_W/1  "PHI_Aircon_Resi3_W"

== system EV_thermal_charger_2015a_jmaab_Can02/Vehicle/CATH/CATH_PNT/HVAC/PTC_Heater1 ==
  note: エアコン用PTCヒーター
      | 熱容量
  P_PTC_Heater_Power : Inport
  Temp_ini : Inport  Port=2
  V_PTC_Heater1_V : Inport  Port=3
  PHI_PTC_Heater1_W : Inport  Port=4
  K->degC : Subsystem
  PTC_Heater : Subsystem
  PTC_Heater_Heat_Capacity : Subsystem
  T_PTC_Heater_degC : Outport
  T_PTC_Heater1_K : Outport  Port=2
  I_PTC_Heater1_A : Outport  Port=3
  wires:
  PTC_Heater_Heat_Capacity/2(T_PTC_Heater3_K) -> PTC_Heater/3(T_PTC_Heater4_K)
  PTC_Heater_Heat_Capacity/1(T_PTC_Heater2_K) -> T_PTC_Heater1_K/1, K->degC/1(K)  "T_PTC_Heater1_K"
  PHI_PTC_Heater1_W/1 -> PTC_Heater_Heat_Capacity/3(PHI_PTC_Heater2_W)
  Temp_ini/1 -> PTC_Heater_Heat_Capacity/1(Temp_ini)
  K->degC/1(degC) -> T_PTC_Heater_degC/1  "T_PTC_Heater_degC"
  P_PTC_Heater_Power/1 -> PTC_Heater/1(P_PTC_Heater_Power)
  V_PTC_Heater1_V/1 -> PTC_Heater/2(V_PTC_Heater4_V)
  PTC_Heater/2(I_PTC_Heater4_A) -> I_PTC_Heater1_A/1
  PTC_Heater/1(PHI_PTC_Heater4_W) -> PTC_Heater_Heat_Capacity/2(PHI_PTC_Heater3_W)

== system EV_thermal_charger_2015a_jmaab_Can02/Vehicle/CATH/CATH_PNT/HVAC/RDCoolant2Air_Heat_Resistance1 ==
  "Aircon_Air_Heat_Resi_KpW " : Inport
  T_Aircon_Air_Resi1_K : Inport  Port=2
  T_Aircon_Air_Resi2_K : Inport  Port=3
  Add : Sum  Inputs=+-
  Divide : Product  Inputs=*/
  Gain : Gain  Gain=-1
  Gain1 : Gain
  PHI_Aircon_Air_Resi1_W : Outport
  PHI_Aircon_Air_Resi2_W : Outport  Port=2
  wires:
  "Aircon_Air_Heat_Resi_KpW "/1 -> Divide/2
  Add/1 -> Divide/1
  Divide/1 -> Gain1/1, Gain/1
  Gain/1 -> PHI_Aircon_Air_Resi2_W/1  "PHI_Aircon_Air_Resi2_W"
  T_Aircon_Air_Resi2_K/1 -> Add/1
  T_Aircon_Air_Resi1_K/1 -> Add/2
  Gain1/1 -> PHI_Aircon_Air_Resi1_W/1  "PHI_Aircon_Air_Resi1_W"

== system EV_thermal_charger_2015a_jmaab_Can02/Vehicle/CATH/CATH_PNT/Seat_Heater/K->degC ==
  K : Inport
  Constant2 : Constant  Value=K2degC
  Sum : Sum  Inputs=++|
  degC : Outport
  wires:
  K/1 -> Sum/2
  Constant2/1 -> Sum/1
  Sum/1 -> degC/1

== system EV_thermal_charger_2015a_jmaab_Can02/Vehicle/CATH/CATH_PNT/Seat_Heater/SeatHT_Heat_Capacity ==
  Temp_ini : Inport
  PHI_SeatHT1_W : Inport  Port=2
  PHI_SeatHT2_W : Inport  Port=3
  Add : Sum
  Add1 : Sum
  Constant : Constant  Value=CATH_PNT_Seat_Heater_Capa_JpK
  Divide : Product  Inputs=/*
  Integrator : Integrator
  degC->K : Subsystem
  T_SeatHT2_K : Outport
  T_SeatHT1_K : Outport  Port=2
  wires:
  PHI_SeatHT2_W/1 -> Add/2
  PHI_SeatHT1_W/1 -> Add/1
  Constant/1 -> Divide/1
  Add/1 -> Divide/2
  Divide/1 -> Integrator/1
  Temp_ini/1 -> degC->K/1(degC)
  Integrator/1 -> Add1/2
  Add1/1 -> T_SeatHT1_K/1, T_SeatHT2_K/1
  degC->K/1(K) -> Add1/1

== system EV_thermal_charger_2015a_jmaab_Can02/Vehicle/CATH/CATH_PNT/Seat_Heater/Seat_HT ==
  P_Seat_Heater_Power : Inport
  V_Seat_HT_V : Inport  Port=2
  T_Seat_HT_K : Inport  Port=3
  Divide_0wari : METI_Lib_vehicle_model/Divide_0wari
  Gain : Gain  Gain=-1
  Terminator : Terminator
  PHI_Seat_HT_W : Outport
  I_Seat_HT_A : Outport  Port=2
  wires:
  P_Seat_Heater_Power/1 -> PHI_Seat_HT_W/1, Divide_0wari/1
  V_Seat_HT_V/1 -> Divide_0wari/2
  Divide_0wari/1 -> Gain/1
  Gain/1 -> I_Seat_HT_A/1  "I_Seat_HT_A"
  T_Seat_HT_K/1 -> Terminator/1

== system EV_thermal_charger_2015a_jmaab_Can02/Vehicle/CATH/CATH_PNT/Seat_Heater/Seat_Heater_Heat_Resistance ==
  T_SeatHT_Resi2_K : Inport
  T_SeatHT_Resi1_K : Inport  Port=2
  Add : Sum  Inputs=+-
  Constant : Constant  Value=CATH_PNT_CABIN_SeatHT_Heat_Resi_KpW
  Divide : Product  Inputs=*/
  Gain : Gain  Gain=-1
  Gain1 : Gain
  PHI_SeatHT_Resi1_W : Outport
  PHI_SeatHT_Resi2_W : Outport  Port=2
  wires:
  Constant/1 -> Divide/2
  Add/1 -> Divide/1
  Divide/1 -> Gain1/1, Gain/1
  Gain/1 -> PHI_SeatHT_Resi2_W/1
  T_SeatHT_Resi2_K/1 -> Add/1
  T_SeatHT_Resi1_K/1 -> Add/2
  Gain1/1 -> PHI_SeatHT_Resi1_W/1

== system EV_thermal_charger_2015a_jmaab_Can02/Vehicle/CNT/CATH_CNT/CATH_CNT/Calc_Temp_Blowout ==
  tSetting_T_User_set_temp_degC : Inport
  T_ATM_PNT_Outside_degC : Inport  Port=2
  T_CABA_PNT_T : Inport  Port=3
  v_VL_PNT_kmph : Inport  Port=4
  Add : Sum
  Constant : Constant  Value=CATH_PNT_CABIN_AIR_Heat_Capa_JpK
  Divide : Product  Inputs=*/
  FB : Subsystem
  FF1 : Subsystem
  Gain : Gain  Gain=0.05
  Subtract : Sum  Inputs=-+
  Subtract1 : Sum  Inputs=+-
  T_blowout_degC : Outport
  T_diff_temp_degC : Outport  Port=2
  wires:
  T_CABA_PNT_T/1 -> FF1/2(T_CABIN_AIR_temp_degC), Subtract/2
  T_ATM_PNT_Outside_degC/1 -> FF1/1(T_Outside_temp_degC)
  Add/1 -> Divide/1
  Divide/1 -> Subtract1/2, T_blowout_degC/1
  Constant/1 -> Gain/1
  Subtract/1 -> Subtract1/1, FB/1(T_diff_temp_degC)
  tSetting_T_User_set_temp_degC/1 -> Subtract/1
  Subtract1/1 -> T_diff_temp_degC/1
  FB/1(Q_FB) -> Add/1
  Gain/1 -> Divide/2
  v_VL_PNT_kmph/1 -> FF1/3(v_VL_PNT_kmph)
  FF1/1(Q_Heat_Transfar) -> Add/2

== system EV_thermal_charger_2015a_jmaab_Can02/Vehicle/CNT/CATH_CNT/CATH_CNT/P_Heatpomp_Power_tgt_calc ==
  note: A/CフラグがON かつ Auto Wind ONの時はヒートポンプ稼働
  T_diff_temp_degC : Inport
  T_AC_PNT_Indoor_degC : Inport  Port=2
  Flag_Aircon : Inport  Port=3
  Flag_AutoWind : Inport  Port=4
  Abs : Abs
  Compare To Constant : simulink/Logic and Bit Operations/Compare To Constant  relop=>  const=0.5  OutDataTypeStr=boolean
  Compare To Constant1 : simulink/Logic and Bit Operations/Compare To Constant  relop=>  const=0.5  OutDataTypeStr=boolean
  Constant : Constant  Value=CATH_CNT_P_Gain_Aircon
  Constant1 : Constant  Value=CATH_CNT_P_Aircon_W_UL
  Constant2 : Constant  Value=CATH_CNT_P_Aircon_W_LL
  Constant3 : Constant  Value=0
  Gain1 : Gain  Gain=-1
  Logical Operator : Logic  AllPortsSameDT=off  OutDataTypeStr=boolean
  Product : Product
  Saturation Dynamic : simulink/Discontinuities/Saturation Dynamic  OutMin=[]  OutMax=[]  OutDataTypeStr=Inherit: Same as second input  OutDataType=fixdt(1, 16)  OutScaling=2^-10  DoSatur=off
  Subtract : Sum
  Switch : Switch  Criteria=u2 > Threshold
  T_Aircon_Indoor_tgt : Lookup_n-D  NumberOfTableDimensions=1  BreakpointsForDimension1=CATH_CNT_T_Aircon_Indoor_degC_x_T_blowout_degC  BeginIndexSearchUsingPreviousIndexResult=on  Table=CATH_CNT_T_Aircon_Indoor_degC  ExtrapMethod=Clip  InternalRulePriority=Speed  RndMeth=Simplest  InputSameDT=on
  V_RDFan_tgt1 : Lookup_n-D  NumberOfTableDimensions=1  BreakpointsForDimension1=CATH_CNT_V_RDFan_x_P_Aircon_W  BeginIndexSearchUsingPreviousIndexResult=on  Table=CATH_CNT_V_RDFan_V  ExtrapMethod=Clip  UseLastTableValue=on  InternalRulePriority=Speed  RndMeth=Simplest  InputSameDT=on
  P_CATH_CNT_Heatpomp_W : Outport
  req_V_CATH_CNT_RDFan_V : Outport  Port=2
  wires:
  T_diff_temp_degC/1 -> T_Aircon_Indoor_tgt/1
  T_Aircon_Indoor_tgt/1 -> Subtract/1
  T_AC_PNT_Indoor_degC/1 -> Gain1/1
  Subtract/1 -> Product/1
  Constant/1 -> Product/2
  Product/1 -> Saturation Dynamic/2
  Constant1/1 -> Saturation Dynamic/1
  Constant2/1 -> Saturation Dynamic/3
  Flag_Aircon/1 -> Compare To Constant/1
  Saturation Dynamic/1 -> Switch/1
  Logical Operator/1 -> Switch/2
  Constant3/1 -> Switch/3
  Switch/1 -> Abs/1, P_CATH_CNT_Heatpomp_W/1
  V_RDFan_tgt1/1 -> req_V_CATH_CNT_RDFan_V/1
  Flag_AutoWind/1 -> Compare To Constant1/1
  Compare To Constant/1 -> Logical Operator/1
  Compare To Constant1/1 -> Logical Operator/2
  Gain1/1 -> Subtract/2
  Abs/1 -> V_RDFan_tgt1/1

== system EV_thermal_charger_2015a_jmaab_Can02/Vehicle/CNT/CATH_CNT/CATH_CNT/P_PTC_Heater_tgt_calc ==
  note: エアコンフラグがONの時は
      | PTCヒーターは使用しない
  note: ヒーター温度が上限値を超過した場合に
      | ヒーター出力を下げる制御
  note: A/CフラグがOFF かつ Auto Wind ONの時
      | PTCヒーターを使用
  T_ATM_PNT_Outside_degC : Inport
  T_PTC_PNT_degC : Inport  Port=2
  Flag_Aircon : Inport  Port=3
  Flag_AutoWind : Inport  Port=4
  Add : Sum
  Compare To Constant : simulink/Logic and Bit Operations/Compare To Constant  relop=>  const=0.5  OutDataTypeStr=boolean
  Compare To Constant1 : simulink/Logic and Bit Operations/Compare To Constant  relop=>  const=0.5  OutDataTypeStr=boolean
  Constant : Constant  Value=CATH_CNT_P_Gain_PTC_Heater
  Constant1 : Constant  Value=CATH_CNT_P_PTC_Heater_W_UL
  Constant2 : Constant  Value=CATH_CNT_P_PTC_Heater_W_LL
  Constant3 : Constant  Value=CATH_CNT_T_PTC_Heater_degC_UL
  Constant4 : Constant  Value=0
  Constant5 : Constant  Value=-inf
  Constant6 : Constant  Value=0
  Logical Operator : Logic  Operator=NOT  AllPortsSameDT=off  OutDataTypeStr=boolean
  Logical Operator1 : Logic  AllPortsSameDT=off  OutDataTypeStr=boolean
  P_PTC_Heater_tgt : Lookup_n-D  NumberOfTableDimensions=1  BreakpointsForDimension1=CATH_CNT_P_PTC_Heater_x_T_Outside_temp_degC  BeginIndexSearchUsingPreviousIndexResult=on  Table=CATH_CNT_P_PTC_Heater  ExtrapMethod=Clip  InternalRulePriority=Speed  RndMeth=Simplest  InputSameDT=on
  Product : Product
  Saturation Dynamic : simulink/Discontinuities/Saturation Dynamic  OutMin=[]  OutMax=[]  OutDataTypeStr=Inherit: Same as second input  OutDataType=fixdt(1, 16)  OutScaling=2^-10  DoSatur=off
  Saturation Dynamic1 : simulink/Discontinuities/Saturation Dynamic  OutMin=[]  OutMax=[]  OutDataTypeStr=Inherit: Same as second input  OutDataType=fixdt(1, 16)  OutScaling=2^-10  DoSatur=off
  Subtract : Sum  Inputs=+-
  Switch : Switch  Criteria=u2 > Threshold
  P_CATH_CNT_PTC_Heater_W : Outport
  wires:
  T_ATM_PNT_Outside_degC/1 -> P_PTC_Heater_tgt/1
  Subtract/1 -> Saturation Dynamic1/2
  Constant/1 -> Product/2
  Add/1 -> Saturation Dynamic/2
  Constant1/1 -> Saturation Dynamic/1
  Constant2/1 -> Saturation Dynamic/3
  T_PTC_PNT_degC/1 -> Subtract/2
  Saturation Dynamic/1 -> Switch/1
  Constant3/1 -> Subtract/1
  Saturation Dynamic1/1 -> Product/1
  Constant4/1 -> Saturation Dynamic1/1
  Constant5/1 -> Saturation Dynamic1/3
  P_PTC_Heater_tgt/1 -> Add/1
  Product/1 -> Add/2
  Flag_Aircon/1 -> Compare To Constant/1
  Compare To Constant/1 -> Logical Operator/1
  Constant6/1 -> Switch/3
  Switch/1 -> P_CATH_CNT_PTC_Heater_W/1
  Logical Operator1/1 -> Switch/2
  Compare To Constant1/1 -> Logical Operator1/2
  Flag_AutoWind/1 -> Compare To Constant1/1
  Logical Operator/1 -> Logical Operator1/1

== system EV_thermal_charger_2015a_jmaab_Can02/Vehicle/CNT/CATH_CNT/CATH_CNT/Subsystem1 ==
  tSetting_P_Charger : Inport
  Compare To Zero : simulink/Logic and Bit Operations/Compare To Zero  relop=>  OutDataTypeStr=boolean
  Constant1 : Constant
  Constant3 : Constant  Value=0
  Switch : Switch  Criteria=u2 > Threshold
  Switch1 : Switch  Criteria=u2 > Threshold
  Flag_Aircon : Outport
  Flag_AutoWind : Outport  Port=2
  wires:
  Switch/1 -> Flag_Aircon/1
  Switch1/1 -> Flag_AutoWind/1
  Compare To Zero/1 -> Switch1/2, Switch/2
  tSetting_P_Charger/1 -> Compare To Zero/1
  Constant3/1 -> Switch1/1, Switch/1
  Constant1/1 -> Switch1/3, Switch/3

== system EV_thermal_charger_2015a_jmaab_Can02/Vehicle/CNT/CATH_CNT/CATH_CNT/T_SeatHT_Temp_tgt_calc ==
  T_diff_temp_degC : Inport
  T_SH_PNT_degC : Inport  Port=2
  Constant : Constant  Value=CATH_CNT_P_Gain_SeatHT
  Constant1 : Constant  Value=CATH_CNT_P_SeatHT_W_UL
  Constant2 : Constant  Value=CATH_CNT_P_SeatHT_W_LL
  Product : Product
  Saturation Dynamic : simulink/Discontinuities/Saturation Dynamic  OutMin=[]  OutMax=[]  OutDataTypeStr=Inherit: Same as second input  OutDataType=fixdt(1, 16)  OutScaling=2^-10  DoSatur=off
  Subtract : Sum  Inputs=+-
  T_SeatHT_Temp_tgt : Lookup_n-D  NumberOfTableDimensions=1  BreakpointsForDimension1=CATH_CNT_T_SeatHT_Temp_degC_x_T_blowout_degC  BeginIndexSearchUsingPreviousIndexResult=on  Table=CATH_CNT_T_SeatHT_Temp_degC  ExtrapMethod=Clip  InternalRulePriority=Speed  RndMeth=Simplest  InputSameDT=on
  P_CATH_CNT_SeatHT_W : Outport
  wires:
  T_diff_temp_degC/1 -> T_SeatHT_Temp_tgt/1
  Subtract/1 -> Product/1
  Constant/1 -> Product/2
  Product/1 -> Saturation Dynamic/2
  Constant1/1 -> Saturation Dynamic/1
  Constant2/1 -> Saturation Dynamic/3
  T_SeatHT_Temp_tgt/1 -> Subtract/1
  T_SH_PNT_degC/1 -> Subtract/2
  Saturation Dynamic/1 -> P_CATH_CNT_SeatHT_W/1

== system EV_thermal_charger_2015a_jmaab_Can02/Vehicle/CNT/CATH_CNT/CATH_CNT/V_HVAC_Fan_calc ==
  T_diff_temp_degC : Inport
  Flag_AutoWind_ON : Inport  Port=2
  Compare To Constant1 : simulink/Logic and Bit Operations/Compare To Constant  relop=>  const=0.5  OutDataTypeStr=boolean
  Constant : Constant  Value=0
  Switch : Switch  Criteria=u2 > Threshold  Threshold=0.5
  V_HVAC_Fan : Lookup_n-D  NumberOfTableDimensions=1  BreakpointsForDimension1=CATH_CNT_V_HVAC_Fan_x_T_blowout_degC  BeginIndexSearchUsingPreviousIndexResult=on  Table=CATH_CNT_V_HVAC_Fan  ExtrapMethod=Clip  InternalRulePriority=Speed  RndMeth=Simplest  InputSameDT=on
  V_CATH_CNT_Aircon_Fan_V : Outport
  wires:
  T_diff_temp_degC/1 -> V_HVAC_Fan/1
  V_HVAC_Fan/1 -> Switch/1
  Flag_AutoWind_ON/1 -> Compare To Constant1/1
  Constant/1 -> Switch/3
  Switch/1 -> V_CATH_CNT_Aircon_Fan_V/1
  Compare To Constant1/1 -> Switch/2

== system EV_thermal_charger_2015a_jmaab_Can02/Vehicle/CNT/CHG_CNT/CHG_CNT/Charge_Current_calc ==
  note: 0：接続ネゴシエーション
      | 1：初期充電
      | 2：本充電
  Charge_mode : Inport
  V_CHG_PNT_Charge_V : Inport  Port=2
  SOC_BT_Hi_PNT_per : Inport  Port=3
  Maximum_Hi_Batt_SOC : Inport  Port=4
  Constant : Constant  Value=P_Charger
  Constant4 : Constant  Value=CHG_CNT_Initial_Charge_Current_A
  Constant5 : Constant  Value=CHG_CNT_Maximum_Charge_Current_A
  Constant6 : Constant  Value=CHG_CNT_Maximum_Charge_Power_W
  Constant7 : Constant  Value=CHG_CNT_Maximum_Charge_Voltage_V
  If : If  IfExpression=u1 < 0.5  ElseIfExpressions=u1 < 1.5
  Initial_Charge : Subsystem  TreatAsAtomicUnit=on
  Manual Switch : ManualSwitch
  Merge : Merge  Inputs=3
  Negotiation_time : Subsystem  TreatAsAtomicUnit=on
  Normal_Charge : Subsystem  TreatAsAtomicUnit=on
  Current_tgt : Outport
  wires:
  Manual Switch/1 -> Normal_Charge/2(Maximum_Charge_Power_W)
  Constant7/1 -> Normal_Charge/3(Maximum_Charge_Voltage_V)
  Negotiation_time/1(Out1) -> Merge/1
  Constant4/1 -> Initial_Charge/1(In1)
  Charge_mode/1 -> If/1
  Constant5/1 -> Normal_Charge/1(Maximum_Charge_Current_A)
  If/2 -> Initial_Charge/Action
  If/1 -> Negotiation_time/Action
  Initial_Charge/1(Out1) -> Merge/2
  If/3 -> Normal_Charge/Action
  Merge/1 -> Current_tgt/1
  Normal_Charge/1(Current_tgt) -> Merge/3
  V_CHG_PNT_Charge_V/1 -> Normal_Charge/4(Battery_Voltage_V)
  SOC_BT_Hi_PNT_per/1 -> Normal_Charge/5(SOC_HiBatt)
  Maximum_Hi_Batt_SOC/1 -> Normal_Charge/6(Maximum_Hi_Batt_SOC)
  Constant/1 -> Manual Switch/2
  Constant6/1 -> Manual Switch/1

== system EV_thermal_charger_2015a_jmaab_Can02/Vehicle/CNT/CHG_CNT/CHG_CNT/Current_rate_limitter ==
  Current_tgt_In1 : Inport
  SOC_BT_Hi_PNT_per : Inport  Port=2
  SOC_UL : Inport  Port=3
  Compare To Zero : simulink/Logic and Bit Operations/Compare To Zero  relop=<  OutDataTypeStr=boolean
  Constant10 : Constant  Value=CHG_CNT_charge_current_rate_UL
  Constant11 : Constant  Value=CHG_CNT_charge_current_rate_LL
  Constant9 : Constant  Value=0
  Rate Limiter Dynamic : simulink/Discontinuities/Rate Limiter Dynamic
  Subtract : Sum  Inputs=+-
  Switch : Switch  Criteria=u2 > Threshold
  tgt_I_CHG_CNT_Charge_A : Outport
  wires:
  Constant11/1 -> Rate Limiter Dynamic/3
  Constant9/1 -> Switch/3
  Rate Limiter Dynamic/1 -> tgt_I_CHG_CNT_Charge_A/1
  Subtract/1 -> Compare To Zero/1
  Switch/1 -> Rate Limiter Dynamic/2
  Compare To Zero/1 -> Switch/2
  Constant10/1 -> Rate Limiter Dynamic/1
  SOC_UL/1 -> Subtract/2
  SOC_BT_Hi_PNT_per/1 -> Subtract/1
  Current_tgt_In1/1 -> Switch/1

== system EV_thermal_charger_2015a_jmaab_Can02/Vehicle/CNT/CHG_CNT/CHG_CNT/counter ==
  note: カウントした数値＞設定数値となったら
      | 1を出力
  note: signal=1でカウントスタート
      | time stepの数字を毎ステップ加算していく
      | signal=0でリセット
  signal : Inport
  time_step : Inport  Port=2
  count_time : Inport  Port=3
  Add : Sum
  Constant : Constant  Value=0
  Constant1 : Constant  Value=0
  Constant2 : Constant
  Memory : Memory
  Product : Product
  Subtract : Sum  Inputs=+-
  Switch : Switch  Criteria=u2 > Threshold  Threshold=0.5
  Switch1 : Switch  Criteria=u2 > Threshold
  Out1 : Outport
  wires:
  signal/1 -> Product/1, Switch/2
  Product/1 -> Add/1
  time_step/1 -> Product/2
  Constant/1 -> Switch/3
  Memory/1 -> Switch/1
  Add/1 -> Memory/1, Subtract/1
  Switch/1 -> Add/2
  count_time/1 -> Subtract/2
  Subtract/1 -> Switch1/2
  Switch1/1 -> Out1/1
  Constant1/1 -> Switch1/3
  Constant2/1 -> Switch1/1

== system EV_thermal_charger_2015a_jmaab_Can02/Vehicle/CNT/CHG_CNT/CHG_CNT/counter1 ==
  note: カウントした数値＞設定数値となったら
      | 1を出力
  note: signal=1でカウントスタート
      | time stepの数字を毎ステップ加算していく
      | signal=0でリセット
  signal : Inport
  time_step : Inport  Port=2
  count_time : Inport  Port=3
  Add : Sum
  Constant : Constant  Value=0
  Constant1 : Constant  Value=0
  Constant2 : Constant
  Memory : Memory
  Product : Product
  Subtract : Sum  Inputs=+-
  Switch : Switch  Criteria=u2 > Threshold  Threshold=0.5
  Switch1 : Switch  Criteria=u2 > Threshold
  Out1 : Outport
  wires:
  signal/1 -> Product/1, Switch/2
  Product/1 -> Add/1
  time_step/1 -> Product/2
  Constant/1 -> Switch/3
  Memory/1 -> Switch/1
  Add/1 -> Memory/1, Subtract/1
  Switch/1 -> Add/2
  count_time/1 -> Subtract/2
  Subtract/1 -> Switch1/2
  Switch1/1 -> Out1/1
  Constant1/1 -> Switch1/3
  Constant2/1 -> Switch1/1
